simulink model "linear_state_estimator"  (R2020b)
settings: Solver=VariableStepAuto  StartTime=0.0  StopTime=10.0  RelTol=1e-3
values from neighbouring files (symbols this model uses):
  A = [-3  -4; 2  1]    [lin_state_estimator.mat]    (also in online_estimator.mat = [-0.25  3; -5  0])
  B = [1 0]    [lin_state_estimator.mat]
  C = [1 3]    [lin_state_estimator.mat]
  D = 0    [lin_state_estimator.mat]
  K = [3 5]    [lin_state_estimator.mat]
  L = [33.8 -3.6]    [lin_state_estimator.mat]
  z0 = 0    [lin_state_estimator.mat]
settings Model: Creator=Prajwal  LastModifiedBy=Prajwal
settings DataIOCC: ReturnWorkspaceOutputs=off

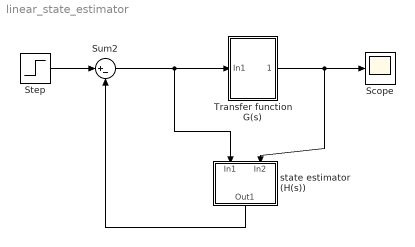
== system linear_state_estimator ==
  Scope : Scope
  Step : Step  Time=0  SampleTime=0
  Sum2 : Sum  Inputs=|+-
  Transfer function G(s) : Subsystem
  state estimator (H(s)) : Subsystem
  wires:
  Sum2/1 -> state estimator (H(s))/1(In1), Transfer function G(s)/1(In1)
  Transfer function G(s)/1(Out1) -> Scope/1, state estimator (H(s))/2(In2)
  state estimator (H(s))/1(Out1) -> Sum2/2
  Step/1 -> Sum2/1

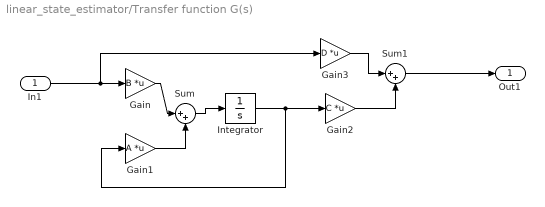
== system linear_state_estimator/Transfer function G(s) ==
  In1 : Inport
  Gain : Gain  Gain=B  Multiplication=Matrix(K*u)
  Gain1 : Gain  Gain=A  Multiplication=Matrix(K*u)
  Gain2 : Gain  Gain=C  Multiplication=Matrix(K*u)
  Gain3 : Gain  Gain=D  Multiplication=Matrix(K*u)
  Integrator : Integrator
  Sum : Sum  Inputs=|++
  Sum1 : Sum  Inputs=|++
  Out1 : Outport
  wires:
  Sum1/1 -> Out1/1
  Sum/1 -> Integrator/1
  Gain2/1 -> Sum1/2
  Gain3/1 -> Sum1/1
  In1/1 -> Gain3/1, Gain/1
  Gain/1 -> Sum/1
  Integrator/1 -> Gain1/1, Gain2/1
  Gain1/1 -> Sum/2

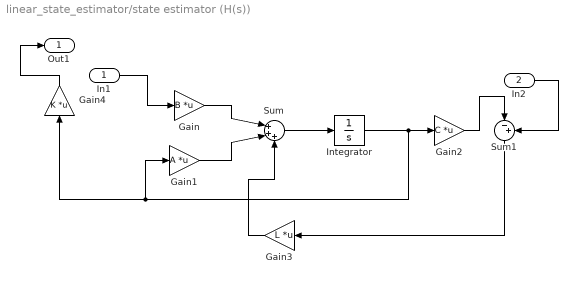
== system linear_state_estimator/state estimator (H(s)) ==
  In1 : Inport
  In2 : Inport  Port=2
  Gain : Gain  Gain=B  Multiplication=Matrix(K*u)
  Gain1 : Gain  Gain=A  Multiplication=Matrix(K*u)
  Gain2 : Gain  Gain=C  Multiplication=Matrix(K*u)
  Gain3 : Gain  Gain=L  Multiplication=Matrix(K*u)
  Gain4 : Gain  Gain=K  Multiplication=Matrix(K*u)
  Integrator : Integrator  InitialCondition=z0
  Sum : Sum  Inputs=|+++
  Sum1 : Sum  Inputs=|-+
  Out1 : Outport
  wires:
  Sum1/1 -> Gain3/1
  Gain2/1 -> Sum1/1
  Gain1/1 -> Sum/2
  Integrator/1 -> Gain2/1, Gain4/1, Gain1/1
  Gain3/1 -> Sum/3
  Sum/1 -> Integrator/1
  Gain/1 -> Sum/1
  In2/1 -> Sum1/2
  In1/1 -> Gain/1
  Gain4/1 -> Out1/1
